simulink model "Ball_Detection"  (R2020a)
settings: Solver=VariableStepAuto  StartTime=0.0  StopTime=inf  RelTol=1e-3
undefined symbols (not defined in the file or in its folder): none, videoinput
libraries: visiontextngfix x1, imaqlib x1, visionsinks x1
settings Model: Creator=vince  LastModifiedBy=vince

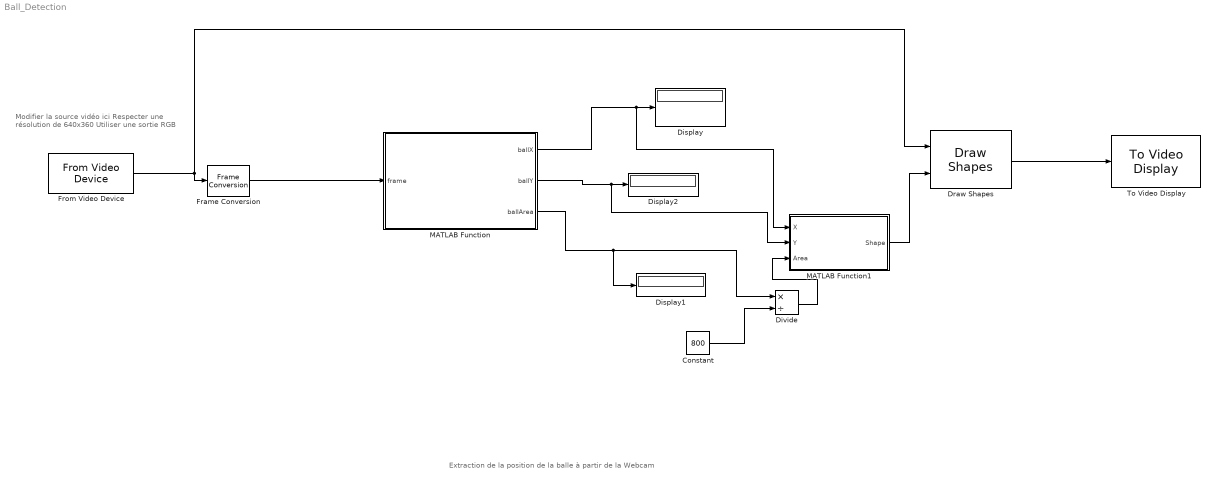
== system Ball_Detection ==
  note: Modifier la source vidéo ici
      | Respecter une résolution de 640x360
      | Utiliser une sortie RGB
  note: Extraction de la position de la balle à partir de la Webcam
  Constant : Constant  Value=800
  Display : Display
  Display1 : Display
  Display2 : Display
  Divide : Product  Inputs=*/
  Draw Shapes : visiontextngfix/Draw Shapes  shape=Circles  fill=on  lineWidth=1  fillClrSource=Specify via dialog  display=User-specified value  intensity=200  color=[255 255 000]  opacity=0.6  viewport=Entire image  antialiasing=off  inType=Obsolete  imagePorts=One multidimensional signal  roundingMode=Floor  overflowMode=off  memoryMode=Specify word length  memoryWordLength=16  prodOutputMode=Binary point scaling  prodOutputWordLength=32  prodOutputFracLength=14  memoryFracLength=15
  Frame Conversion : FrameConversion  OutFrame=Sample-based
  From Video Device : imaqlib/From Video Device  DeviceMenu=winvideo 1 (Microsoft® LifeCam HD-3000)  Device=winvideo 1 (Microsoft® LifeCam HD-3000)  ObjConstructor=videoinput('winvideo', 1)  VideoFormatMenu=YUY2_640x360  VideoFormat=YUY2_640x360  VideoSource=input1  ROIPosition=[0 0 360 640]  EnableHWTrigger=off  TriggerConfiguration=none/none  SampleTime=1/30  OutputPortsMode=One multidimensional signal  DataType=single  CanDoHWTrigger=no  ReturnedColorSpace=rgb  BlockHandle=32.0001  ROIWidth=640  ROIHeight=360  ROIColumn=0  ROIRow=0  EngXMLPath=C:\Program Files\MATLAB\R2020a\toolbox\imaq\imaq\private  DevXMLPath=C:\ProgramData\MATLAB\SupportPackages\R2020a\toolbox\imaq\supportpackages\genericvideo\adaptor\win64  EngLibPath=C:\Program Files\MATLAB\R2020a\toolbox\imaq\imaqblks\imaqmex\win64  ColorSpace=rgb  BayerSensorAlignment=grbg  ImaqMode=off
  MATLAB Function : MATLAB Function  TreatAsAtomicUnit=on  RTWFcnName=detectOrangeBall
  MATLAB Function1 : MATLAB Function  TreatAsAtomicUnit=on
  To Video Display : visionsinks/To Video Display  windowSizeMode=Normal  openAtMdlStart=on  fullScreen=off  videoWindowX=-355  videoWindowY=194  saveWindowSize=off  videoWindowWidth=1280  videoWindowHeight=720  inputColorFormat=RGB  inputType=Obsolete  imagePorts=One multidimensional signal  OutputDevice=On-screen video monitor  dataOrg=Column-major  isWindowOpen=off
  wires:
  Frame Conversion/1 -> MATLAB Function/1(frame)
  From Video Device/1 -> Frame Conversion/1, Draw Shapes/1
  MATLAB Function/1(ballX) -> MATLAB Function1/1(X), Display/1
  MATLAB Function/3(ballArea) -> Divide/1, Display1/1
  Draw Shapes/1 -> To Video Display/1
  MATLAB Function/2(ballY) -> MATLAB Function1/2(Y), Display2/1
  MATLAB Function1/1(Shape) -> Draw Shapes/2
  Constant/1 -> Divide/2
  Divide/1 -> MATLAB Function1/3(Area)

== matlab function Ball_Detection/MATLAB Function1 ==
  data: X input size=[2]; Shape output size=[1 3]; Y input size=[2]; Area input size=[2]
function Shape = Concatenate(X,Y ,Area)
Shape=[int32(X(1)), int32(Y(1)), int32(Area(1))];

== matlab function Ball_Detection/MATLAB Function ==
  data: ballX output size=[2]; ballY output size=[2]; frame input; ballArea output size=[2]
function [ballX, ballY, ballArea] = detectOrangeBall(frame)
% Create the default minimum and maximum HSV values for orange color
orangeMin = [0.05 0.4 0.5];
orangeMax = [0.15 1.0 1.0];
ballArea = int32(0); % Fixed size for Simulink

% Create a blob analysis object
blobAnalyzer = vision.BlobAnalysis('MinimumBlobArea', 100, 'MaximumBlobArea', 10000);

while true
    % Check if the input frame is empty
    if isempty(frame)
        ballX = NaN;
        ballY = NaN;
        ballArea = int32(0)
        break;
    end
    
    % Convert the frame to HSV color space
    hsv = rgb2hsv(frame);
    
    % Create a mask for the orange color
    mask = (hsv(:,:,1) >= orangeMin(1)) & (hsv(:,:,1) <= orangeMax(1)) & ...
           (hsv(:,:,2) >= orangeMin(2)) & (hsv(:,:,2) <= orangeMax(2)) & ...
           (hsv(:,:,3) >= orangeMin(3)) & (hsv(:,:,3) <= orangeMax(3));
       
    % Perform blob analysis on the mask
    [areas, centroids] = step(blobAnalyzer, mask);
    
    % Find the largest blob in the image
    index = [];
    if ~isempty(areas)
        [~, index] = max(areas);
        ballX = centroids(index, 1);
        ballY = centroids(index, 2);
        ballArea = areas(index);
    else
        ballX = 0;
        ballY = 0;
        ballArea = int32(0)
        break; % No ball has been found
    end
    
    % Output the centroid and area of the largest blob
    if ~isempty(centroids)
        ballX = centroids(index, 1);
        ballY = centroids(index, 2);
        ballArea = areas(index);
        break;
    end
end
